simulink model "Pendulum_Stabilization_Sinusoidal_Cart_Motion"  (R2022b)
settings: Solver=VariableStepAuto  StartTime=0.0  StopTime=20.0  RelTol=1e-3
libraries: slpidlib x1, simulink x1
settings Model: Creator=Shaan Sapru  LastModifiedBy=Shaan Sapru

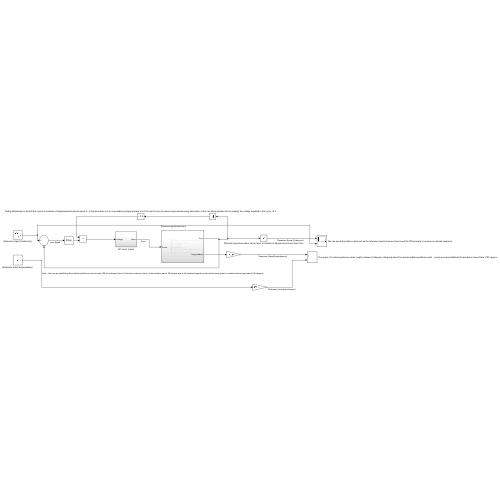
[thumbnail: Simulink's stored preview of the top-level diagram]
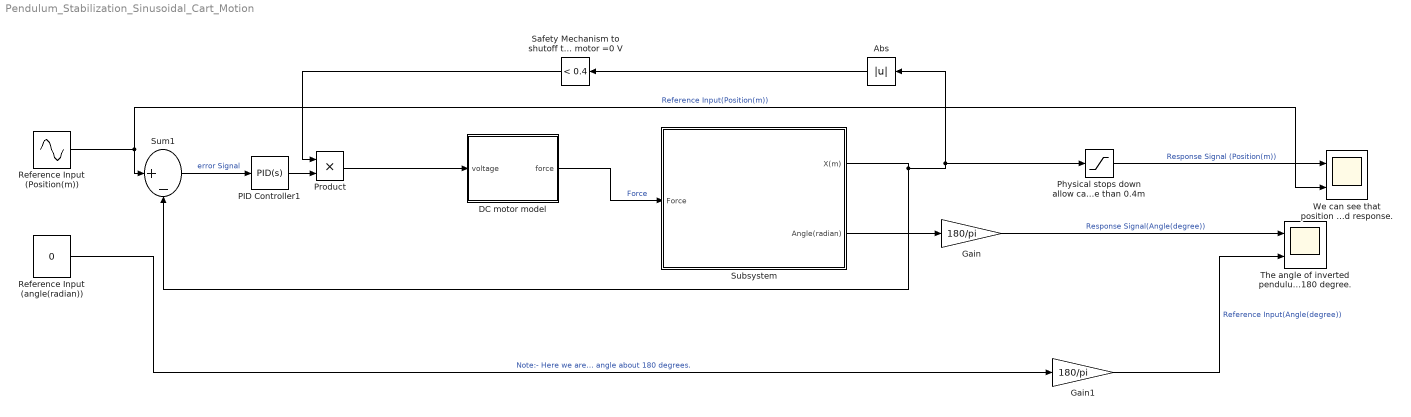
== system Pendulum_Stabilization_Sinusoidal_Cart_Motion ==
  Abs : Abs  SaturateOnIntegerOverflow=off
  DC motor model : Subsystem
  Gain : Gain  Gain=180/pi
  Gain1 : Gain  Gain=180/pi
  PID Controller1 : slpidlib/PID Controller  Controller=PID  Form=Parallel  TimeDomain=Continuous-time  UseExternalTs=off  SampleTime=-1  IntegratorMethod=Forward Euler  FilterMethod=Forward Euler  ControllerParametersSource=internal  P=-21.7778359586833  I=-0.726120198049073  UseKiTs=off  D=-28.7223003489043  N=0.697092906180596  UseFilter=on  TunerSelectOption=Transfer Function Based (PID Tuner App)  InitialConditionSource=internal  InitialConditionForIntegrator=0  InitialConditionForFilter=0  DifferentiatorICPrevScaledInput=0  ExternalReset=none  TrackingMode=off  Kt=1  LimitOutput=off  SatLimitsSource=internal  UpperSaturationLimit=inf  LowerSaturationLimit=-inf  LinearizeAsGain=on  AntiWindupMode=none  Kb=1  LimitIntegrator=off  UpperIntegratorSaturationLimit=inf  LowerIntegratorSaturationLimit=-inf  POutMin=[]  POutMax=[]  IOutMin=[]  IOutMax=[]  DOutMin=[]  DOutMax=[]  NOutMin=[]  NOutMax=[]  SumOutMin=[]  SumOutMax=[]  SaturationOutMin=[]  SaturationOutMax=[]  PParamMin=[]  PParamMax=[]  IParamMin=[]  IParamMax=[]  DParamMin=[]  DParamMax=[]  NParamMin=[]  NParamMax=[]  KbParamMin=[]  KbParamMax=[]  KtParamMin=[]  KtParamMax=[]  KbOutMin=[]  KbOutMax=[]  KtOutMin=[]  KtOutMax=[]  IntegratorOutMin=[]  IntegratorOutMax=[]  FilterOutMin=[]  FilterOutMax=[]  SumI1OutMin=[]  SumI1OutMax=[]  SumI2OutMin=[]  SumI2OutMax=[]  SumI3OutMin=[]  SumI3OutMax=[]  SumI4OutMin=[]  SumI4OutMax=[]  SumDOutMin=[]  SumDOutMax=[]  DifferentiatorOutMin=[]  DifferentiatorOutMax=[]  FilterDiffOutCoefMin=[]  FilterDiffOutCoefMax=[]  ReciprocalOutMin=[]  ReciprocalOutMax=[]  SumDenOutMin=[]  SumDenOutMax=[]  SumNumOutMin=[]  SumNumOutMax=[]  DivideOutMin=[]  DivideOutMax=[]  UdiffTsProdOutMin=[]  UdiffTsProdOutMax=[]  NTsProdOutMin=[]  NTsProdOutMax=[]  UintegralTsProdOutMin=[]  UintegralTsProdOutMax=[]  UngainTsProdOutMin=[]  UngainTsProdOutMax=[]  ClampingZeroOutDataTypeStr=Inherit: Inherit via back propagation  ClampingZeroOutMin=[]  ClampingZeroOutMax=[]  FilterDenConstantOutDataTypeStr=Inherit: Inherit via back propagation  FilterDenConstantOutMin=[]  FilterDenConstantOutMax=[]  PCopyOutDataTypeStr=Inherit: Inherit via back propagation  PCopyOutMin=[]  PCopyOutMax=[]  NCopyOutDataTypeStr=Inherit: Inherit via back propagation  NCopyOutMin=[]  NCopyOutMax=[]  IntegratorContinuousStateAttributes=''  IntegratorStateMustResolveToSignalObject=off  IntegratorRTWStateStorageClass=Auto  FilterContinuousStateAttributes=''  FilterStateMustResolveToSignalObject=off  FilterRTWStateStorageClass=Auto  ParallelPVariant=InternalParameters  IdealPVariant=Disabled  IVariant=InternalParameters  DVariant=InternalParameters  IntegratorVariant=Continuous  SatVariant=Disabled  AWVariant=Passthrough  PCopyVariant=Disabled  TRVariant=Disabled  FdbkBlocksVariant=Forward  IdealPFdbkVariant=Disabled  SatFdbkVariant=Disabled  DerivativeFilterVariant=ContFilter  NVariant=InternalParameters  NCopyVariant=Disabled  FilterICVariant=InternalICsFilter  IntegratorICVariant=InternalICs  ExternalResetVariant=Disabled  TRSumVariant=Passthrough  SumFdbkVariant=Disabled  SumVariant=Sum_PID  TsampFilterVariant=InternalTs  TsampNgainVariant=Passthrough  TsampIntegralVariant=Passthrough  ExternalSaturationOutDataTypeStr=Inherit: Same as second input
  Physical stops down allow cart to have a modulus of displacement more than 0.4m : Saturate  UpperLimit=0.4  LowerLimit=-0.4
  Product : Product
  Reference Input (Position(m)) : Sin  Amplitude=0.3  SampleTime=0
  "Reference Input (angle(radian)) " : Constant  Value=0
  Safety Mechanism to shutoff the system if modulus of displacement becomes equal to  0.4m(more than 0.4 is not possible as physical stops at x=0.4m which here has been respresented using saturation) of the cart about position=0m by making the voltage supplied to the motor =0 V : simulink/Logic and Bit Operations/Compare To Constant  relop=<  const=0.4  OutDataTypeStr=boolean
  Subsystem : Subsystem
  Sum1 : Sum  Inputs=|+-
  "The angle of inverted pendulum varies roughly between [-6degree,+6degree] about the desired stable equilibrium point  , hence we have stabilised the pendulum about theta =180 degree." : Scope  NumInputPorts=2
  We can see that position varies just as the reference input hence we have tuned the PID properly to ensure our desired response. : Scope  NumInputPorts=2
  wires:
  Sum1/1 -> PID Controller1/1  "error Signal"
  Subsystem/1(X(m)) -> Sum1/2, Physical stops down allow cart to have a modulus of displacement more than 0.4m/1, Abs/1
  Reference Input (Position(m))/1 -> Sum1/1, We can see that position varies just as the reference input hence we have tuned the PID properly to ensure our desired response./2  "Reference Input(Position(m))"
  "Reference Input (angle(radian)) "/1 -> Gain1/1  "Note:- Here we are stabilising about stable equilibrium point of angle 180 but reference Input is 0 because reference Input  is the deviation about 180 degree and in the linearised equations also which were given to us theta was the angle about 180 degrees."
  DC motor model/1(force) -> Subsystem/1(Force)  "Force"
  Subsystem/2(Angle(radian)) -> Gain/1
  PID Controller1/1 -> Product/2
  Gain/1 -> "The angle of inverted pendulum varies roughly between [-6degree,+6degree] about the desired stable equilibrium point  , hence we have stabilised the pendulum about theta =180 degree."/1  "Response Signal(Angle(degree))"
  Gain1/1 -> "The angle of inverted pendulum varies roughly between [-6degree,+6degree] about the desired stable equilibrium point  , hence we have stabilised the pendulum about theta =180 degree."/2  "Reference Input(Angle(degree))"
  Safety Mechanism to shutoff the system if modulus of displacement becomes equal to  0.4m(more than 0.4 is not possible as physical stops at x=0.4m which here has been respresented using saturation) of the cart about position=0m by making the voltage supplied to the motor =0 V/1 -> Product/1
  Product/1 -> DC motor model/1(voltage)
  Abs/1 -> Safety Mechanism to shutoff the system if modulus of displacement becomes equal to  0.4m(more than 0.4 is not possible as physical stops at x=0.4m which here has been respresented using saturation) of the cart about position=0m by making the voltage supplied to the motor =0 V/1
  Physical stops down allow cart to have a modulus of displacement more than 0.4m/1 -> We can see that position varies just as the reference input hence we have tuned the PID properly to ensure our desired response./1  "Response Signal (Position(m))"

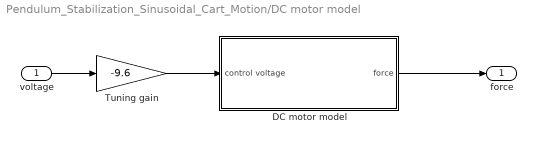
== system Pendulum_Stabilization_Sinusoidal_Cart_Motion/DC motor model ==
  voltage : Inport
  DC motor model : Subsystem  mask{J=0.0000140, Kt=0.05, Kb=0.05, d=0.000001, R=2.5, L=0.0025}
      mask prompts: J "Moment of inertia"; Kt "Torque constant"; Kb "Electromotive force constant"; d "Linear approximation of viscous friction"; R "Electrical circuit resistance"; L "Electrical circuit inductance"
      mask Display: disp('DC motor')
  Tuning gain : Gain  Gain=-9.6
  force : Outport
  wires:
  Tuning gain/1 -> DC motor model/1(control voltage)
  voltage/1 -> Tuning gain/1
  DC motor model/1(force) -> force/1

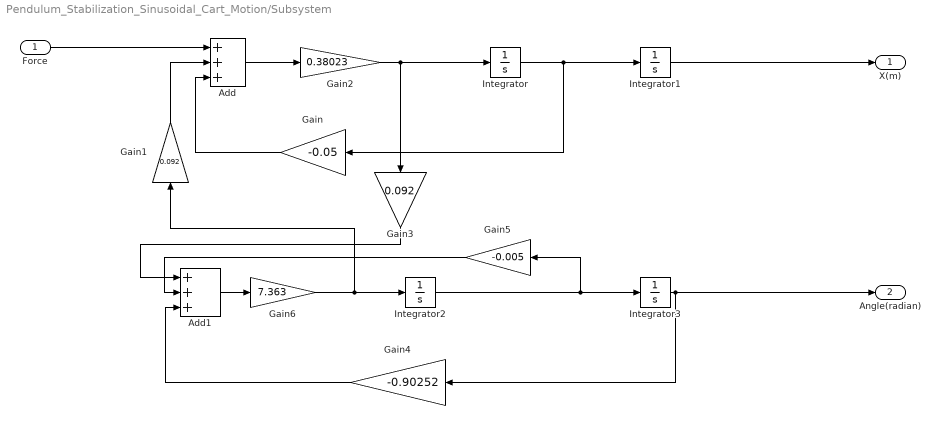
== system Pendulum_Stabilization_Sinusoidal_Cart_Motion/Subsystem ==
  Force : Inport
  Add : Sum  Inputs=+++
  Add1 : Sum  Inputs=+++
  Gain : Gain  Gain=-0.05
  Gain1 : Gain  Gain=0.092
  Gain2 : Gain  Gain=0.38023
  Gain3 : Gain  Gain=0.092
  Gain4 : Gain  Gain=-0.90252
  Gain5 : Gain  Gain=-0.005
  Gain6 : Gain  Gain=7.363
  Integrator : Integrator  InitialCondition=0.0
  Integrator1 : Integrator
  Integrator2 : Integrator
  Integrator3 : Integrator
  X(m) : Outport
  Angle(radian) : Outport  Port=2
  wires:
  Gain1/1 -> Add/2
  Integrator2/1 -> Gain5/1, Integrator3/1
  Integrator3/1 -> Gain4/1, Angle(radian)/1
  Gain2/1 -> Gain3/1, Integrator/1
  Add1/1 -> Gain6/1
  Gain4/1 -> Add1/3
  Gain/1 -> Add/3
  Integrator1/1 -> X(m)/1
  Integrator/1 -> Gain/1, Integrator1/1
  Force/1 -> Add/1
  Add/1 -> Gain2/1
  Gain3/1 -> Add1/1
  Gain5/1 -> Add1/2
  Gain6/1 -> Integrator2/1, Gain1/1

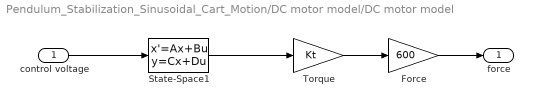
== system Pendulum_Stabilization_Sinusoidal_Cart_Motion/DC motor model/DC motor model ==
  control voltage : Inport
  Force : Gain  Gain=600
  State-Space1 : StateSpace  A=[-d/J Kt/J;-Kb/L -R/L]  B=[0; 1/L]  C=[0 1]  D=0  InitialCondition=0
  Torque : Gain  Gain=Kt
  force : Outport
  wires:
  control voltage/1 -> State-Space1/1
  State-Space1/1 -> Torque/1
  Torque/1 -> Force/1
  Force/1 -> force/1
